simulink model "Model_14Bus_Microgrid_R2018"  (R2018b)
settings: Solver=ode23tb  StartTime=0.0  StopTime=0.35  MaxStep=1e-2  RelTol=1e-3
InitFcn:
  | Set_parameters_R2018
StopFcn:
  | Save_Data;
  | Graphics;
values from neighbouring files (symbols this model uses):
  Clink = Ceq*2    (= 0.217013888889)    [Set_parameters_R2017b.m]    (also in Set_parameters_R2018.m)
  dis1 = 0.15    [Set_parameters_R2017b.m]    (also in Set_parameters_R2018.m)
  dis10 = 6    [Set_parameters_R2017b.m]    (also in Set_parameters_R2018.m)
  dis11 = 3    [Set_parameters_R2017b.m]    (also in Set_parameters_R2018.m)
  dis12 = 6    [Set_parameters_R2017b.m]    (also in Set_parameters_R2018.m)
  dis13 = 3    [Set_parameters_R2017b.m]    (also in Set_parameters_R2018.m)
  dis14 = 2    [Set_parameters_R2017b.m]    (also in Set_parameters_R2018.m)
  dis2 = 0.2    [Set_parameters_R2017b.m]    (also in Set_parameters_R2018.m)
  dis3 = 0.15    [Set_parameters_R2017b.m]    (also in Set_parameters_R2018.m)
  dis4 = 0.4    [Set_parameters_R2017b.m]    (also in Set_parameters_R2018.m)
  dis5 = 0.4    [Set_parameters_R2017b.m]    (also in Set_parameters_R2018.m)
  dis6 = 0.4    [Set_parameters_R2017b.m]    (also in Set_parameters_R2018.m)
  dis7 = 0.1    [Set_parameters_R2017b.m]    (also in Set_parameters_R2018.m)
  dis8 = 2    [Set_parameters_R2017b.m]    (also in Set_parameters_R2018.m)
  dis9 = 6    [Set_parameters_R2017b.m]    (also in Set_parameters_R2018.m)
  Fc = 33 * Fnom    (= 1980)    [Set_parameters_R2017b.m]    (also in Set_parameters_R2018.m)
  Fnom = 60    [Main_DC_MG.m]    (also in Set_parameters_R2017b.m; Set_parameters_R2018.m)
  Increment_MPPT = 0.01    [Set_parameters_R2017b.m]    (also in Set_parameters_R2018.m)
  Ki_Ireg = 20    [Set_parameters_R2017b.m]    (also in Set_parameters_R2018.m)
  Ki_VDCreg = 400    [Set_parameters_R2017b.m]    (also in Set_parameters_R2018.m)
  Kp_Ireg = 0.3    [Set_parameters_R2017b.m]    (also in Set_parameters_R2018.m)
  Kp_VDCreg = 2    [Set_parameters_R2017b.m]    (also in Set_parameters_R2018.m)
  LimitL_Ireg = -1.5    [Set_parameters_R2017b.m]    (also in Set_parameters_R2018.m)
  LimitL_VDCreg = -1.5    [Set_parameters_R2017b.m]    (also in Set_parameters_R2018.m)
  Limits_MPPT = [ 583 357 ]    [Set_parameters_R2017b.m]    (also in Set_parameters_R2018.m)
  LimitU_Ireg = 1.5    [Set_parameters_R2017b.m]    (also in Set_parameters_R2018.m)
  LimitU_VDCreg = 1.5    [Set_parameters_R2017b.m]    (also in Set_parameters_R2018.m)
  P_Load_2 = S_Load_2* PF_Load_2    (= 36000)    [Set_parameters_R2017b.m]    (also in Set_parameters_R2018.m)
  P_Load_3 = S_Load_3* PF_Load_3    (= 25500)    [Set_parameters_R2017b.m]    (also in Set_parameters_R2018.m)
  Pnom = 1e6    (= 1000000)    [Set_parameters_R2017b.m]    (also in Set_parameters_R2018.m)
  Pnom_T1 = 1.5e6    (= 1500000)    [Set_parameters_R2017b.m]    (also in Set_parameters_R2018.m)
  Pnom_T2 = 1.5e6    (= 1500000)    [Set_parameters_R2017b.m]    (also in Set_parameters_R2018.m)
  Pnom_T3 = 4e6    (= 4000000)    [Set_parameters_R2017b.m]    (also in Set_parameters_R2018.m)
  Pnom_xfo = Pnom    (= 1000000)    [Set_parameters_R2017b.m]    (also in Set_parameters_R2018.m)
  Ql_Load_2 = S_Load_2 * sin(acos(PF_Load_2))    [Set_parameters_R2017b.m]    (also in Set_parameters_R2018.m)
  Ql_Load_3 = S_Load_3 * sin(acos(PF_Load_3))    [Set_parameters_R2017b.m]    (also in Set_parameters_R2018.m)
  R_Load_9 = (Vnom_prim * 1.35)^2 / P_Load_9    (= 1084.6153125)    [Set_parameters_R2017b.m]    (also in Set_parameters_R2018.m)
  R_Load_DC = Vnom_DC^2/ P_Load_DC    (= 45)    [Main_DC_MG.m]    (also in Set_parameters_R2017b.m; Set_parameters_R2018.m)
  Rl = 0.394    [Set_parameters_R2017b.m]    (also in Set_parameters_R2018.m)
  Rls = 0.198    [Set_parameters_R2017b.m]    (also in Set_parameters_R2018.m)
  Ts = Ts_Power    (= 5.05050505051e-06)    [Main_DC_MG.m]    (also in Set_parameters_R2017b.m; Set_parameters_R2018.m)
  Ts_Control = 10*Ts_Power    (= 5.05050505051e-05)    [Main_DC_MG.m]    (also in Set_parameters_R2017b.m; Set_parameters_R2018.m)
  Ts_Power = 1/(33*Fnom)/100    (= 5.05050505051e-06)    [Main_DC_MG.m]    (also in Set_parameters_R2017b.m; Set_parameters_R2018.m)
  V1_LL_T3 = 69e3    (= 69000)    [Set_parameters_R2017b.m]    (also in Set_parameters_R2018.m)
  Vf = 0    [Set_parameters_R2017b.m]    (also in Set_parameters_R2018.m)
  Vfd = 0    [Set_parameters_R2017b.m]    (also in Set_parameters_R2018.m)
  Vnom_DC = 300    [Main_DC_MG.m]    (also in Set_parameters_R2017b.m; Set_parameters_R2018.m)
  Vnom_dc = 480    [Set_parameters_R2017b.m]    (also in Set_parameters_R2018.m)
  Vnom_Diesel = 2.4e3    (= 2400)    [Set_parameters_R2017b.m]    (also in Set_parameters_R2018.m)
  Vnom_prim = 13.8e3    (= 13800)    [Set_parameters_R2017b.m]    (also in Set_parameters_R2018.m)
  Vnom_sec = 220    [Set_parameters_R2017b.m]    (also in Set_parameters_R2018.m)
  Vnom_ter_AC_DC = 150    [Set_parameters_R2017b.m]    (also in Set_parameters_R2018.m)
  Xl = 0.1168    [Set_parameters_R2017b.m]    (also in Set_parameters_R2018.m)
  Xls = 0.1089    [Set_parameters_R2017b.m]    (also in Set_parameters_R2018.m)
undefined symbols (not defined in the file or in its folder): D1, Delta, Hydride, Ion, Lithium, max_min, Metal, Nickel, RL, RLff, sigbuilder_block
libraries: powerlib x202, powerlib_meascontrol x152, simulink x14, powerlib_extras x14, electricdrivelib x4, re_lib x2
(part 6 of 10)

== system Model_14Bus_Microgrid_R2018/Bus_7/Power Factor Block1 ==
  Vabc : Inport
  Iabc : Inport  Port=2
  Complex to Magnitude-Angle : ComplexToMagnitudeAngle
  Conv pu2 : Gain  Gain=sqrt (3) /Vnom_prim  SaturateOnIntegerOverflow=on  OutDataTypeStr=Inherit: Same as input  ParamDataTypeStr=Inherit: Same as input
  Mux : Mux  Inputs=2
  Mux1 : Mux  Inputs=2
  Power : powerlib_meascontrol/Measurements/Power  Freq=Freq  Vinit=Vinit  Iinit=Iinit  Ts=Ts
      settings: SourceProductName=Simscape Electrical
  RMS3 : powerlib_meascontrol/Measurements/RMS  TrueRMS=on  Freq=60  RMSInit=0  Ts=0
      settings: SourceProductName=Simscape Electrical
  RMS4 : powerlib_meascontrol/Measurements/RMS  TrueRMS=on  Freq=60  RMSInit=0  Ts=0
      settings: SourceProductName=Simscape Electrical
  Real-Imag to Complex : RealImagToComplex
  Terminator : Terminator
  compara : Gain  SaturateOnIntegerOverflow=on  OutDataTypeStr=Inherit: Same as input  ParamDataTypeStr=Inherit: Same as input
  cos(theta) : Trigonometry  Operator=cos
  to Kw : Gain  Gain=1/1000
  to Kw1 : Gain  Gain=1/1000
  Pabc : Outport
  Qabc : Outport  Port=2
  Vabc y Vabc (rms) : Outport  Port=3
  Iabc y Iabc (rms) : Outport  Port=4
  "PFabc " : Outport  Port=5
  tag scope: P_abc_Bus7=global, Q_abc_Bus7=global, Vabc_LL_pu_Bus7=global
  wires:
  Complex to Magnitude-Angle/2 -> cos(theta)/1
  Real-Imag to Complex/1 -> Complex to Magnitude-Angle/1
  cos(theta)/1 -> "PFabc "/1
  Complex to Magnitude-Angle/1 -> Terminator/1
  Iabc/1 -> RMS4/1, compara/1, Power/2
  RMS4/1 -> Mux1/2
  Mux1/1 -> Iabc y Iabc (rms)/1
  Mux/1 -> Vabc y Vabc (rms)/1
  Vabc/1 -> Power/1, Mux/2, RMS3/1
  compara/1 -> Mux1/1
  Conv pu2/1 -> [Vabc_LL_pu_Bus7]
  RMS3/1 -> Conv pu2/1, Mux/1
  Power/2 -> Qabc/1, Real-Imag to Complex/2, to Kw/1
  Power/1 -> to Kw1/1, Pabc/1, Real-Imag to Complex/1
  to Kw/1 -> [Q_abc_Bus7]
  to Kw1/1 -> [P_abc_Bus7]

== system Model_14Bus_Microgrid_R2018/Bus_8      /PLL ==
  Vabc_LN_pu : Inport
  2pi60'1 : Constant  Value=2*pi*60
  2pi60'2 : Constant  Value=2*pi*60
  2pi60'3 : Constant  Value=2*pi*60
  Constant : Constant  Value=90
  Demux : Demux  Outputs=3
  Gain1 : Gain  Gain=180/pi  SaturateOnIntegerOverflow=on  OutDataTypeStr=Inherit: Same as input  ParamDataTypeStr=Inherit: Same as input
  Gain2 : Gain  Gain=180/pi  SaturateOnIntegerOverflow=on  OutDataTypeStr=Inherit: Same as input  ParamDataTypeStr=Inherit: Same as input
  Gain3 : Gain  Gain=180/pi  SaturateOnIntegerOverflow=on  OutDataTypeStr=Inherit: Same as input  ParamDataTypeStr=Inherit: Same as input
  Mux : Mux  Inputs=3
  Pll1 : Subsystem
  Pll2 : Subsystem
  Pll3 : Subsystem
  Sum : Sum  Inputs=|++
  delta_abc : Outport
  wires:
  Vabc_LN_pu/1 -> Demux/1
  Demux/1 -> Pll3/1(señal)
  2pi60'3/1 -> Pll3/2(w)
  Pll3/1(f cos (rad)) -> Gain1/1
  Demux/2 -> Pll1/1(señal)
  2pi60'1/1 -> Pll1/2(w)
  Gain2/1 -> Mux/2
  Demux/3 -> Pll2/1(señal)
  2pi60'2/1 -> Pll2/2(w)
  Pll2/1(f cos (rad)) -> Gain3/1
  Gain3/1 -> Mux/3
  Pll1/1(f cos (rad)) -> Gain2/1
  Mux/1 -> Sum/1
  Gain1/1 -> Mux/1
  Constant/1 -> Sum/2
  Sum/1 -> delta_abc/1

== system Model_14Bus_Microgrid_R2018/Bus_8      /Power Factor Block1 ==
  Vabc : Inport
  Iabc : Inport  Port=2
  Complex to Magnitude-Angle : ComplexToMagnitudeAngle
  Conv pu2 : Gain  Gain=sqrt (3) /Vnom_Diesel  SaturateOnIntegerOverflow=on  OutDataTypeStr=Inherit: Same as input  ParamDataTypeStr=Inherit: Same as input
  Gain : Gain  Gain=-1/1000
  Gain1 : Gain  Gain=-1/1000
  Mux : Mux  Inputs=2
  Mux1 : Mux  Inputs=2
  Power : powerlib_meascontrol/Measurements/Power  Freq=Freq  Vinit=Vinit  Iinit=Iinit  Ts=Ts
      settings: SourceProductName=Simscape Electrical
  RMS3 : powerlib_meascontrol/Measurements/RMS  TrueRMS=on  Freq=60  RMSInit=0  Ts=0
      settings: SourceProductName=Simscape Electrical
  RMS4 : powerlib_meascontrol/Measurements/RMS  TrueRMS=on  Freq=60  RMSInit=0  Ts=0
      settings: SourceProductName=Simscape Electrical
  Real-Imag to Complex : RealImagToComplex
  Terminator : Terminator
  compara : Gain  SaturateOnIntegerOverflow=on  OutDataTypeStr=Inherit: Same as input  ParamDataTypeStr=Inherit: Same as input
  cos(theta) : Trigonometry  Operator=cos
  Pabc : Outport
  Qabc : Outport  Port=2
  Vabc y Vabc (rms) : Outport  Port=3
  Iabc y Iabc (rms) : Outport  Port=4
  "PFabc " : Outport  Port=5
  tag scope: P_abc_Bus8=global, Q_abc_Bus8=global, Vabc_LL_pu_Bus8=global
  wires:
  Complex to Magnitude-Angle/2 -> cos(theta)/1
  Real-Imag to Complex/1 -> Complex to Magnitude-Angle/1
  cos(theta)/1 -> "PFabc "/1
  Complex to Magnitude-Angle/1 -> Terminator/1
  Iabc/1 -> RMS4/1, compara/1, Power/2
  RMS4/1 -> Mux1/2
  Mux1/1 -> Iabc y Iabc (rms)/1
  Mux/1 -> Vabc y Vabc (rms)/1
  Vabc/1 -> Power/1, Mux/2, RMS3/1
  compara/1 -> Mux1/1
  Conv pu2/1 -> [Vabc_LL_pu_Bus8]
  RMS3/1 -> Conv pu2/1, Mux/1
  Power/2 -> Qabc/1, Real-Imag to Complex/2, Gain/1
  Power/1 -> Gain1/1, Pabc/1, Real-Imag to Complex/1
  Gain/1 -> [Q_abc_Bus8]
  Gain1/1 -> [P_abc_Bus8]

== system Model_14Bus_Microgrid_R2018/Bus_9/PLL ==
  Vabc_LN_pu : Inport
  2pi60'1 : Constant  Value=2*pi*60
  2pi60'2 : Constant  Value=2*pi*60
  2pi60'3 : Constant  Value=2*pi*60
  Constant : Constant  Value=90
  Demux : Demux  Outputs=3
  Gain1 : Gain  Gain=180/pi  SaturateOnIntegerOverflow=on  OutDataTypeStr=Inherit: Same as input  ParamDataTypeStr=Inherit: Same as input
  Gain2 : Gain  Gain=180/pi  SaturateOnIntegerOverflow=on  OutDataTypeStr=Inherit: Same as input  ParamDataTypeStr=Inherit: Same as input
  Gain3 : Gain  Gain=180/pi  SaturateOnIntegerOverflow=on  OutDataTypeStr=Inherit: Same as input  ParamDataTypeStr=Inherit: Same as input
  Mux : Mux  Inputs=3
  Pll1 : Subsystem
  Pll2 : Subsystem
  Pll3 : Subsystem
  Sum : Sum  Inputs=|++
  delta_abc : Outport
  wires:
  Vabc_LN_pu/1 -> Demux/1
  Demux/1 -> Pll3/1(señal)
  2pi60'3/1 -> Pll3/2(w)
  Pll3/1(f cos (rad)) -> Gain1/1
  Demux/2 -> Pll1/1(señal)
  2pi60'1/1 -> Pll1/2(w)
  Gain2/1 -> Mux/2
  Demux/3 -> Pll2/1(señal)
  2pi60'2/1 -> Pll2/2(w)
  Pll2/1(f cos (rad)) -> Gain3/1
  Gain3/1 -> Mux/3
  Pll1/1(f cos (rad)) -> Gain2/1
  Mux/1 -> Sum/1
  Gain1/1 -> Mux/1
  Constant/1 -> Sum/2
  Sum/1 -> delta_abc/1

== system Model_14Bus_Microgrid_R2018/Bus_9/Power Factor Block1 ==
  Vabc : Inport
  Iabc : Inport  Port=2
  Complex to Magnitude-Angle : ComplexToMagnitudeAngle
  Conv pu2 : Gain  Gain=sqrt (3) /Vnom_prim  SaturateOnIntegerOverflow=on  OutDataTypeStr=Inherit: Same as input  ParamDataTypeStr=Inherit: Same as input
  Mux : Mux  Inputs=2
  Mux1 : Mux  Inputs=2
  Power : powerlib_meascontrol/Measurements/Power  Freq=Freq  Vinit=Vinit  Iinit=Iinit  Ts=Ts
      settings: SourceProductName=Simscape Electrical
  RMS3 : powerlib_meascontrol/Measurements/RMS  TrueRMS=on  Freq=60  RMSInit=0  Ts=0
      settings: SourceProductName=Simscape Electrical
  RMS4 : powerlib_meascontrol/Measurements/RMS  TrueRMS=on  Freq=60  RMSInit=0  Ts=0
      settings: SourceProductName=Simscape Electrical
  Real-Imag to Complex : RealImagToComplex
  Terminator : Terminator
  compara : Gain  SaturateOnIntegerOverflow=on  OutDataTypeStr=Inherit: Same as input  ParamDataTypeStr=Inherit: Same as input
  cos(theta) : Trigonometry  Operator=cos
  to Kw : Gain  Gain=1/1000
  to Kw1 : Gain  Gain=1/1000
  Pabc : Outport
  Qabc : Outport  Port=2
  Vabc y Vabc (rms) : Outport  Port=3
  Iabc y Iabc (rms) : Outport  Port=4
  "PFabc " : Outport  Port=5
  tag scope: P_abc_Bus9=global, Q_abc_Bus9=global, Vabc_LL_pu_Bus9=global
  wires:
  Complex to Magnitude-Angle/2 -> cos(theta)/1
  Real-Imag to Complex/1 -> Complex to Magnitude-Angle/1
  cos(theta)/1 -> "PFabc "/1
  Complex to Magnitude-Angle/1 -> Terminator/1
  Iabc/1 -> RMS4/1, compara/1, Power/2
  RMS4/1 -> Mux1/2
  Mux1/1 -> Iabc y Iabc (rms)/1
  Mux/1 -> Vabc y Vabc (rms)/1
  Vabc/1 -> Power/1, Mux/2, RMS3/1
  compara/1 -> Mux1/1
  RMS3/1 -> Conv pu2/1, Mux/1
  Conv pu2/1 -> [Vabc_LL_pu_Bus9]
  Power/2 -> Qabc/1, Real-Imag to Complex/2, to Kw/1
  Power/1 -> to Kw1/1, Pabc/1, Real-Imag to Complex/1
  to Kw/1 -> [Q_abc_Bus9]
  to Kw1/1 -> [P_abc_Bus9]

== system Model_14Bus_Microgrid_R2018/Bus_AC PV /PLL ==
  Vabc_LN_pu : Inport
  2pi60'1 : Constant  Value=2*pi*60
  2pi60'2 : Constant  Value=2*pi*60
  2pi60'3 : Constant  Value=2*pi*60
  Constant : Constant  Value=90
  Demux : Demux  Outputs=3
  Gain1 : Gain  Gain=180/pi  SaturateOnIntegerOverflow=on  OutDataTypeStr=Inherit: Same as input  ParamDataTypeStr=Inherit: Same as input
  Gain2 : Gain  Gain=180/pi  SaturateOnIntegerOverflow=on  OutDataTypeStr=Inherit: Same as input  ParamDataTypeStr=Inherit: Same as input
  Gain3 : Gain  Gain=180/pi  SaturateOnIntegerOverflow=on  OutDataTypeStr=Inherit: Same as input  ParamDataTypeStr=Inherit: Same as input
  Mux : Mux  Inputs=3
  Pll1 : Subsystem
  Pll2 : Subsystem
  Pll3 : Subsystem
  Sum : Sum  Inputs=|++
  delta_abc : Outport
  wires:
  Vabc_LN_pu/1 -> Demux/1
  Demux/1 -> Pll3/1(señal)
  2pi60'3/1 -> Pll3/2(w)
  Pll3/1(f cos (rad)) -> Gain1/1
  Demux/2 -> Pll1/1(señal)
  2pi60'1/1 -> Pll1/2(w)
  Gain2/1 -> Mux/2
  Demux/3 -> Pll2/1(señal)
  2pi60'2/1 -> Pll2/2(w)
  Pll2/1(f cos (rad)) -> Gain3/1
  Gain3/1 -> Mux/3
  Pll1/1(f cos (rad)) -> Gain2/1
  Mux/1 -> Sum/1
  Gain1/1 -> Mux/1
  Constant/1 -> Sum/2
  Sum/1 -> delta_abc/1

== system Model_14Bus_Microgrid_R2018/Bus_AC PV /Power Factor Block1 ==
  Vabc : Inport
  Iabc : Inport  Port=2
  Complex to Magnitude-Angle : ComplexToMagnitudeAngle
  Mux : Mux  Inputs=2
  Mux1 : Mux  Inputs=2
  Power : powerlib_meascontrol/Measurements/Power  Freq=Freq  Vinit=Vinit  Iinit=Iinit  Ts=Ts
      settings: SourceProductName=Simscape Electrical
  RMS3 : powerlib_meascontrol/Measurements/RMS  TrueRMS=on  Freq=60  RMSInit=0  Ts=0
      settings: SourceProductName=Simscape Electrical
  RMS4 : powerlib_meascontrol/Measurements/RMS  TrueRMS=on  Freq=60  RMSInit=0  Ts=0
      settings: SourceProductName=Simscape Electrical
  Real-Imag to Complex : RealImagToComplex
  Terminator : Terminator
  compara : Gain  SaturateOnIntegerOverflow=on  OutDataTypeStr=Inherit: Same as input  ParamDataTypeStr=Inherit: Same as input
  cos(theta) : Trigonometry  Operator=cos
  Pabc : Outport
  Qabc : Outport  Port=2
  Vabc y Vabc (rms) : Outport  Port=3
  Iabc y Iabc (rms) : Outport  Port=4
  "PFabc " : Outport  Port=5
  wires:
  Power/1 -> Pabc/1, Real-Imag to Complex/1
  Power/2 -> Qabc/1, Real-Imag to Complex/2
  Complex to Magnitude-Angle/2 -> cos(theta)/1
  Real-Imag to Complex/1 -> Complex to Magnitude-Angle/1
  cos(theta)/1 -> "PFabc "/1
  Complex to Magnitude-Angle/1 -> Terminator/1
  Iabc/1 -> RMS4/1, compara/1, Power/2
  RMS4/1 -> Mux1/2
  Mux1/1 -> Iabc y Iabc (rms)/1
  Mux/1 -> Vabc y Vabc (rms)/1
  Vabc/1 -> Power/1, Mux/2, RMS3/1
  compara/1 -> Mux1/1
  RMS3/1 -> Mux/1

== system Model_14Bus_Microgrid_R2018/Bus_AC//DC3/Battery system ==
  note: DC Bus
  note: Bettery
  "0 = Enable (Do it after transient, so that it does not calculate ripples during transient) 1 = Reset after every change in current reference" : Constant  Value=0
  Current Inst : Scope
  Current going to/ from the battery : Scope
  Display6 : Display
  Mean : powerlib_meascontrol/Measurements/Mean  Freq=10  Vinit=0  Ts=0
      settings: SourceProductName=Simscape Electrical
  Power : Product
  Power Bess : Scope
  Ripple Calculations : Subsystem
  Ripple in Boost : Display
  Ripple in Buck : Display
  Vbat : Scope
  Vdc : Scope
  to Kw : Gain  Gain=1/1000
  wires:
  to Kw/1 -> Display6/1, Power Bess/1
  Mean/1 -> Power/2
  Power/1 -> to Kw/1
  Ripple Calculations/1(Ripple in Buck) -> Ripple in Buck/1
  "0 = Enable (Do it after transient, so that it does not calculate ripples during transient) 1 = Reset after every change in current reference"/1 -> Ripple Calculations/2(Reset)
  Ripple Calculations/2(Ripple in Boost) -> Ripple in Boost/1
  [Idc_bus] -> Mean/1, Ripple Calculations/1(Signal), Current Inst/1
  [current] -> Current going to/ from the battery/1
  [Vdc_bus] -> Vdc/1, Power/1
  [Vdc_battery] -> Vbat/1

== system Model_14Bus_Microgrid_R2018/Bus_AC//DC3/PV system ==
  note: Bus DC
  note: PV
  Bus Selector : BusSelector  OutputSignals=V_PV,I_PV,I_diode,Irradiance (W/m2),Temperature (deg C)
  Current going to/ DC bus : Scope
  "P (kW) " : Display
      settings: Format=bank  Decimation=2000
  PV : Scope  NumInputPorts=3
  PV1 : Scope  NumInputPorts=5
  Pmean : Subsystem
  Vdc Boost : Display
      settings: Format=bank  Decimation=2000
  Vdc DC bus : Scope
  tag scope: I_PV=global, Idiode_PV=global, Ir=global, Temp=global, V_PV=global
  wires:
  [V_PV] -> PV/1  "V_PV"
  [I_PV] -> PV/2  "I_PV"
  [Idiode_PV] -> PV/3  "Idiode_PV"
  [m_PV] -> Bus Selector/1
  Bus Selector/1 -> [V_PV]  "<V_PV>"
  Bus Selector/2 -> [I_PV]  "<I_PV>"
  Bus Selector/4 -> [Ir]  "<Irradiance (W/m2)>"
  Bus Selector/3 -> [Idiode_PV]  "<I_diode>"
  Bus Selector/5 -> [Temp]  "<Temperature (deg C)>"
  [Temp] -> PV1/2  "Temp (deg. C)"
  [D] -> PV1/5  "Duty Cycle"
  Pmean/2(V) -> Vdc Boost/1, PV1/4  "Vmean (V)"
  [Ir] -> PV1/1  "Ir (W/m^2)"
  Pmean/1(P) -> "P (kW) "/1, PV1/3  "Pmean  (kW)"
  [I_DC_bus_PV] -> Current going to/ DC bus/1
  [V_DC_bus_PV] -> Vdc DC bus/1

== system Model_14Bus_Microgrid_R2018/Bus_AC//DC4/PLL ==
  Vabc_LN_pu : Inport
  2pi60'1 : Constant  Value=2*pi*60
  2pi60'2 : Constant  Value=2*pi*60
  2pi60'3 : Constant  Value=2*pi*60
  Constant : Constant  Value=90
  Demux : Demux  Outputs=3
  Gain1 : Gain  Gain=180/pi  SaturateOnIntegerOverflow=on  OutDataTypeStr=Inherit: Same as input  ParamDataTypeStr=Inherit: Same as input
  Gain2 : Gain  Gain=180/pi  SaturateOnIntegerOverflow=on  OutDataTypeStr=Inherit: Same as input  ParamDataTypeStr=Inherit: Same as input
  Gain3 : Gain  Gain=180/pi  SaturateOnIntegerOverflow=on  OutDataTypeStr=Inherit: Same as input  ParamDataTypeStr=Inherit: Same as input
  Mux : Mux  Inputs=3
  Pll1 : Subsystem
  Pll2 : Subsystem
  Pll3 : Subsystem
  Sum : Sum  Inputs=|++
  delta_abc : Outport
  wires:
  Vabc_LN_pu/1 -> Demux/1
  Demux/1 -> Pll3/1(señal)
  2pi60'3/1 -> Pll3/2(w)
  Pll3/1(f cos (rad)) -> Gain1/1
  Demux/2 -> Pll1/1(señal)
  2pi60'1/1 -> Pll1/2(w)
  Gain2/1 -> Mux/2
  Demux/3 -> Pll2/1(señal)
  2pi60'2/1 -> Pll2/2(w)
  Pll2/1(f cos (rad)) -> Gain3/1
  Gain3/1 -> Mux/3
  Pll1/1(f cos (rad)) -> Gain2/1
  Mux/1 -> Sum/1
  Gain1/1 -> Mux/1
  Constant/1 -> Sum/2
  Sum/1 -> delta_abc/1

== system Model_14Bus_Microgrid_R2018/Bus_AC//DC4/Power Factor Block1 ==
  Vabc : Inport
  Iabc : Inport  Port=2
  Complex to Magnitude-Angle : ComplexToMagnitudeAngle
  Mux : Mux  Inputs=2
  Mux1 : Mux  Inputs=2
  Power : powerlib_meascontrol/Measurements/Power  Freq=Freq  Vinit=Vinit  Iinit=Iinit  Ts=Ts
      settings: SourceProductName=Simscape Electrical
  RMS3 : powerlib_meascontrol/Measurements/RMS  TrueRMS=on  Freq=60  RMSInit=0  Ts=0
      settings: SourceProductName=Simscape Electrical
  RMS4 : powerlib_meascontrol/Measurements/RMS  TrueRMS=on  Freq=60  RMSInit=0  Ts=0
      settings: SourceProductName=Simscape Electrical
  Real-Imag to Complex : RealImagToComplex
  Terminator : Terminator
  compara : Gain  SaturateOnIntegerOverflow=on  OutDataTypeStr=Inherit: Same as input  ParamDataTypeStr=Inherit: Same as input
  cos(theta) : Trigonometry  Operator=cos
  Pabc : Outport
  Qabc : Outport  Port=2
  Vabc y Vabc (rms) : Outport  Port=3
  Iabc y Iabc (rms) : Outport  Port=4
  "PFabc " : Outport  Port=5
  wires:
  Power/1 -> Pabc/1, Real-Imag to Complex/1
  Power/2 -> Qabc/1, Real-Imag to Complex/2
  Complex to Magnitude-Angle/2 -> cos(theta)/1
  Real-Imag to Complex/1 -> Complex to Magnitude-Angle/1
  cos(theta)/1 -> "PFabc "/1
  Complex to Magnitude-Angle/1 -> Terminator/1
  Iabc/1 -> RMS4/1, compara/1, Power/2
  RMS4/1 -> Mux1/2
  Mux1/1 -> Iabc y Iabc (rms)/1
  Mux/1 -> Vabc y Vabc (rms)/1
  Vabc/1 -> Power/1, Mux/2, RMS3/1
  compara/1 -> Mux1/1
  RMS3/1 -> Mux/1

== system Model_14Bus_Microgrid_R2018/Bus_AC//DC5/PLL ==
  Vabc_LN_pu : Inport
  2pi60'1 : Constant  Value=2*pi*60
  2pi60'2 : Constant  Value=2*pi*60
  2pi60'3 : Constant  Value=2*pi*60
  Constant : Constant  Value=90
  Demux : Demux  Outputs=3
  Gain1 : Gain  Gain=180/pi  SaturateOnIntegerOverflow=on  OutDataTypeStr=Inherit: Same as input  ParamDataTypeStr=Inherit: Same as input
  Gain2 : Gain  Gain=180/pi  SaturateOnIntegerOverflow=on  OutDataTypeStr=Inherit: Same as input  ParamDataTypeStr=Inherit: Same as input
  Gain3 : Gain  Gain=180/pi  SaturateOnIntegerOverflow=on  OutDataTypeStr=Inherit: Same as input  ParamDataTypeStr=Inherit: Same as input
  Mux : Mux  Inputs=3
  Pll1 : Subsystem
  Pll2 : Subsystem
  Pll3 : Subsystem
  Sum : Sum  Inputs=|++
  delta_abc : Outport
  wires:
  Vabc_LN_pu/1 -> Demux/1
  Demux/1 -> Pll3/1(señal)
  2pi60'3/1 -> Pll3/2(w)
  Pll3/1(f cos (rad)) -> Gain1/1
  Demux/2 -> Pll1/1(señal)
  2pi60'1/1 -> Pll1/2(w)
  Gain2/1 -> Mux/2
  Demux/3 -> Pll2/1(señal)
  2pi60'2/1 -> Pll2/2(w)
  Pll2/1(f cos (rad)) -> Gain3/1
  Gain3/1 -> Mux/3
  Pll1/1(f cos (rad)) -> Gain2/1
  Mux/1 -> Sum/1
  Gain1/1 -> Mux/1
  Constant/1 -> Sum/2
  Sum/1 -> delta_abc/1

== system Model_14Bus_Microgrid_R2018/Bus_AC//DC5/Power Factor Block1 ==
  Vabc : Inport
  Iabc : Inport  Port=2
  Complex to Magnitude-Angle : ComplexToMagnitudeAngle
  Mux : Mux  Inputs=2
  Mux1 : Mux  Inputs=2
  Power : powerlib_meascontrol/Measurements/Power  Freq=Freq  Vinit=Vinit  Iinit=Iinit  Ts=Ts
      settings: SourceProductName=Simscape Electrical
  RMS3 : powerlib_meascontrol/Measurements/RMS  TrueRMS=on  Freq=60  RMSInit=0  Ts=0
      settings: SourceProductName=Simscape Electrical
  RMS4 : powerlib_meascontrol/Measurements/RMS  TrueRMS=on  Freq=60  RMSInit=0  Ts=0
      settings: SourceProductName=Simscape Electrical
  Real-Imag to Complex : RealImagToComplex
  Terminator : Terminator
  compara : Gain  SaturateOnIntegerOverflow=on  OutDataTypeStr=Inherit: Same as input  ParamDataTypeStr=Inherit: Same as input
  cos(theta) : Trigonometry  Operator=cos
  Pabc : Outport
  Qabc : Outport  Port=2
  Vabc y Vabc (rms) : Outport  Port=3
  Iabc y Iabc (rms) : Outport  Port=4
  "PFabc " : Outport  Port=5
  wires:
  Power/1 -> Pabc/1, Real-Imag to Complex/1
  Power/2 -> Qabc/1, Real-Imag to Complex/2
  Complex to Magnitude-Angle/2 -> cos(theta)/1
  Real-Imag to Complex/1 -> Complex to Magnitude-Angle/1
  cos(theta)/1 -> "PFabc "/1
  Complex to Magnitude-Angle/1 -> Terminator/1
  Iabc/1 -> RMS4/1, compara/1, Power/2
  RMS4/1 -> Mux1/2
  Mux1/1 -> Iabc y Iabc (rms)/1
  Mux/1 -> Vabc y Vabc (rms)/1
  Vabc/1 -> Power/1, Mux/2, RMS3/1
  compara/1 -> Mux1/1
  RMS3/1 -> Mux/1

== system Model_14Bus_Microgrid_R2018/Bus_slack /PLL ==
  Vabc_LN_pu : Inport
  2pi60'1 : Constant  Value=2*pi*60
  2pi60'2 : Constant  Value=2*pi*60
  2pi60'3 : Constant  Value=2*pi*60
  Constant : Constant  Value=90
  Demux : Demux  Outputs=3
  Gain1 : Gain  Gain=180/pi  SaturateOnIntegerOverflow=on  OutDataTypeStr=Inherit: Same as input  ParamDataTypeStr=Inherit: Same as input
  Gain2 : Gain  Gain=180/pi  SaturateOnIntegerOverflow=on  OutDataTypeStr=Inherit: Same as input  ParamDataTypeStr=Inherit: Same as input
  Gain3 : Gain  Gain=180/pi  SaturateOnIntegerOverflow=on  OutDataTypeStr=Inherit: Same as input  ParamDataTypeStr=Inherit: Same as input
  Mux : Mux  Inputs=3
  Pll1 : Subsystem
  Pll2 : Subsystem
  Pll3 : Subsystem
  Sum : Sum  Inputs=|++
  delta_abc : Outport
  wires:
  Vabc_LN_pu/1 -> Demux/1
  Demux/1 -> Pll3/1(señal)
  2pi60'3/1 -> Pll3/2(w)
  Pll3/1(f cos (rad)) -> Gain1/1
  Demux/2 -> Pll1/1(señal)
  2pi60'1/1 -> Pll1/2(w)
  Gain2/1 -> Mux/2
  Demux/3 -> Pll2/1(señal)
  2pi60'2/1 -> Pll2/2(w)
  Pll2/1(f cos (rad)) -> Gain3/1
  Gain3/1 -> Mux/3
  Pll1/1(f cos (rad)) -> Gain2/1
  Mux/1 -> Sum/1
  Gain1/1 -> Mux/1
  Constant/1 -> Sum/2
  Sum/1 -> delta_abc/1

== system Model_14Bus_Microgrid_R2018/Bus_slack /Power Factor Block1 ==
  Vabc : Inport
  Iabc : Inport  Port=2
  Complex to Magnitude-Angle : ComplexToMagnitudeAngle
  Conv pu2 : Gain  Gain=sqrt (3) /Vnom_prim  SaturateOnIntegerOverflow=on  OutDataTypeStr=Inherit: Same as input  ParamDataTypeStr=Inherit: Same as input
  Gain : Gain  Gain=-1/1000
  Gain1 : Gain  Gain=-1/1000
  Mux : Mux  Inputs=2
  Mux1 : Mux  Inputs=2
  Power : powerlib_meascontrol/Measurements/Power  Freq=Freq  Vinit=Vinit  Iinit=Iinit  Ts=Ts
      settings: SourceProductName=Simscape Electrical
  RMS3 : powerlib_meascontrol/Measurements/RMS  TrueRMS=on  Freq=60  RMSInit=0  Ts=0
      settings: SourceProductName=Simscape Electrical
  RMS4 : powerlib_meascontrol/Measurements/RMS  TrueRMS=on  Freq=60  RMSInit=0  Ts=0
      settings: SourceProductName=Simscape Electrical
  Real-Imag to Complex : RealImagToComplex
  Terminator : Terminator
  compara : Gain  SaturateOnIntegerOverflow=on  OutDataTypeStr=Inherit: Same as input  ParamDataTypeStr=Inherit: Same as input
  cos(theta) : Trigonometry  Operator=cos
  Pabc : Outport
  Qabc : Outport  Port=2
  Vabc y Vabc (rms) : Outport  Port=3
  Iabc y Iabc (rms) : Outport  Port=4
  "PFabc " : Outport  Port=5
  tag scope: P_abc_Bus13=global, Q_abc_Bus13=global, Vabc_LL_pu_Bus13=global
  wires:
  Complex to Magnitude-Angle/2 -> cos(theta)/1
  Real-Imag to Complex/1 -> Complex to Magnitude-Angle/1
  cos(theta)/1 -> "PFabc "/1
  Complex to Magnitude-Angle/1 -> Terminator/1
  Iabc/1 -> RMS4/1, compara/1, Power/2
  RMS4/1 -> Mux1/2
  Mux1/1 -> Iabc y Iabc (rms)/1
  Mux/1 -> Vabc y Vabc (rms)/1
  Vabc/1 -> Power/1, Mux/2, RMS3/1
  compara/1 -> Mux1/1
  RMS3/1 -> Conv pu2/1, Mux/1
  Conv pu2/1 -> [Vabc_LL_pu_Bus13]
  Power/1 -> Gain/1, Pabc/1, Real-Imag to Complex/1
  Power/2 -> Qabc/1, Real-Imag to Complex/2, Gain1/1
  Gain1/1 -> [Q_abc_Bus13]
  Gain/1 -> [P_abc_Bus13]

== system Model_14Bus_Microgrid_R2018/Control measurement/measurement ==
  Ground4 : powerlib/Elements/Ground  LConnTagsString=a
      settings: SourceProductName=Simscape Electrical
  Mux1 : Mux  Inputs=3
  Mux2 : Mux  Inputs=3
  Mux7 : Mux  Inputs=3
  Vab : powerlib/Measurements/Voltage Measurement  Tag=PoWeRsYsTeMmEaSuReMeNt  PhasorSimulation=off  OutputType=Magnitude  PSBequivalent=0
      settings: SourceProductName=Simscape Electrical
  Vab{1..3,5} (4 alike) : powerlib_extras/Discrete Measurements/Discrete  RMS value  Freq=60  Mag_Init=0  Ts=Ts_Power
  Vbc : powerlib/Measurements/Voltage Measurement  Tag=PoWeRsYsTeMmEaSuReMeNt  PhasorSimulation=off  OutputType=Magnitude  PSBequivalent=0
      settings: SourceProductName=Simscape Electrical
  Vca : powerlib/Measurements/Voltage Measurement  Tag=PoWeRsYsTeMmEaSuReMeNt  PhasorSimulation=off  OutputType=Magnitude  PSBequivalent=0
      settings: SourceProductName=Simscape Electrical
  a : powerlib/Measurements/Voltage Measurement  Tag=PoWeRsYsTeMmEaSuReMeNt  PhasorSimulation=off  OutputType=Magnitude  PSBequivalent=0
      settings: SourceProductName=Simscape Electrical
  b : powerlib/Measurements/Voltage Measurement  Tag=PoWeRsYsTeMmEaSuReMeNt  PhasorSimulation=off  OutputType=Magnitude  PSBequivalent=0
      settings: SourceProductName=Simscape Electrical
  c : powerlib/Measurements/Voltage Measurement  Tag=PoWeRsYsTeMmEaSuReMeNt  PhasorSimulation=off  OutputType=Magnitude  PSBequivalent=0
      settings: SourceProductName=Simscape Electrical
  A : PMIOPort  Side=Left
  B : PMIOPort  Port=2  Side=Left
  C : PMIOPort  Port=3  Side=Left
  Vph : Outport
  VL-L : Outport  Port=2
  VL-L_rms : Outport  Port=3
  Vph_rms : Outport  Port=4
  wires:
  a/1 -> Mux7/1, Vab5/1
  b/1 -> Mux7/2, Vab1/1
  c/1 -> Mux7/3, Vab2/1
  Mux7/1 -> Vph/1
  Vab/1 -> Mux1/1
  Vbc/1 -> Mux1/2
  Vca/1 -> Mux1/3
  Mux1/1 -> Vab3/1, VL-L/1
  Vab5/1 -> Mux2/1
  Vab1/1 -> Mux2/2
  Vab2/1 -> Mux2/3
  Mux2/1 -> Vph_rms/1
  Vab3/1 -> VL-L_rms/1
  connections:
  Ground4/LConn1 -- c/LConn2 -- b/LConn2 -- a/LConn2
  A/RConn1 -- a/LConn1 -- Vab/LConn1 -- Vca/LConn2
  B/RConn1 -- b/LConn1 -- Vab/LConn2 -- Vbc/LConn1
  C/RConn1 -- c/LConn1 -- Vbc/LConn2 -- Vca/LConn1

== system Model_14Bus_Microgrid_R2018/Control measurement2/measurement2 ==
  Ground4 : powerlib/Elements/Ground  LConnTagsString=a
      settings: SourceProductName=Simscape Electrical
  Mux1 : Mux  Inputs=3
  Mux2 : Mux  Inputs=3
  Mux7 : Mux  Inputs=3
  Vab : powerlib/Measurements/Voltage Measurement  Tag=PoWeRsYsTeMmEaSuReMeNt  PhasorSimulation=off  OutputType=Magnitude  PSBequivalent=0
      settings: SourceProductName=Simscape Electrical
  Vab{1..3,5} (4 alike) : powerlib_extras/Discrete Measurements/Discrete  RMS value  Freq=60  Mag_Init=0  Ts=Ts_Power
  Vbc : powerlib/Measurements/Voltage Measurement  Tag=PoWeRsYsTeMmEaSuReMeNt  PhasorSimulation=off  OutputType=Magnitude  PSBequivalent=0
      settings: SourceProductName=Simscape Electrical
  Vca : powerlib/Measurements/Voltage Measurement  Tag=PoWeRsYsTeMmEaSuReMeNt  PhasorSimulation=off  OutputType=Magnitude  PSBequivalent=0
      settings: SourceProductName=Simscape Electrical
  a : powerlib/Measurements/Voltage Measurement  Tag=PoWeRsYsTeMmEaSuReMeNt  PhasorSimulation=off  OutputType=Magnitude  PSBequivalent=0
      settings: SourceProductName=Simscape Electrical
  b : powerlib/Measurements/Voltage Measurement  Tag=PoWeRsYsTeMmEaSuReMeNt  PhasorSimulation=off  OutputType=Magnitude  PSBequivalent=0
      settings: SourceProductName=Simscape Electrical
  c : powerlib/Measurements/Voltage Measurement  Tag=PoWeRsYsTeMmEaSuReMeNt  PhasorSimulation=off  OutputType=Magnitude  PSBequivalent=0
      settings: SourceProductName=Simscape Electrical
  A : PMIOPort  Side=Left
  B : PMIOPort  Port=2  Side=Left
  C : PMIOPort  Port=3  Side=Left
  Vph : Outport
  VL-L : Outport  Port=2
  VL-L_rms : Outport  Port=3
  Vph_rms : Outport  Port=4
  wires:
  a/1 -> Mux7/1, Vab5/1
  b/1 -> Mux7/2, Vab1/1
  c/1 -> Mux7/3, Vab2/1
  Mux7/1 -> Vph/1
  Vab/1 -> Mux1/1
  Vbc/1 -> Mux1/2
  Vca/1 -> Mux1/3
  Mux1/1 -> Vab3/1, VL-L/1
  Vab5/1 -> Mux2/1
  Vab1/1 -> Mux2/2
  Vab2/1 -> Mux2/3
  Mux2/1 -> Vph_rms/1
  Vab3/1 -> VL-L_rms/1
  connections:
  Ground4/LConn1 -- c/LConn2 -- b/LConn2 -- a/LConn2
  A/RConn1 -- a/LConn1 -- Vab/LConn1 -- Vca/LConn2
  B/RConn1 -- b/LConn1 -- Vab/LConn2 -- Vbc/LConn1
  C/RConn1 -- c/LConn1 -- Vbc/LConn2 -- Vca/LConn1

== system Model_14Bus_Microgrid_R2018/DATA  ADQUISITION/Delta_abc ==
  Mux3 : Mux  Inputs=14
  f3 : ToWorkspace  VariableName=ang_abc  SaveFormat=Timeseries  SampleTime=-1
  wires:
  [delta_abc_Bus10] -> Mux3/10
  [delta_abc_Bus4] -> Mux3/4
  [delta_abc_Bus7] -> Mux3/7
  [delta_abc_Bus8] -> Mux3/8
  [delta_abc_Bus11] -> Mux3/11
  [delta_abc_Bus5] -> Mux3/5
  [delta_abc_Bus9] -> Mux3/9
  [delta_abc_Bus2] -> Mux3/2
  [delta_abc_Bus1] -> Mux3/1
  [delta_abc_Bus12] -> Mux3/12
  [delta_abc_Bus14] -> Mux3/14
  Mux3/1 -> f3/1
  [delta_abc_Bus6] -> Mux3/6
  [delta_abc_Bus13] -> Mux3/13
  [delta_abc_Bus3] -> Mux3/3

== system Model_14Bus_Microgrid_R2018/DATA  ADQUISITION/PF_abc ==
  Mux2 : Mux  Inputs=14
  f3 : ToWorkspace  VariableName=PF_abc  SaveFormat=Timeseries  SampleTime=-1
  wires:
  [PFabc_Bus2] -> Mux2/2
  [PFabc_Bus4] -> Mux2/4
  [PFabc_Bus1] -> Mux2/1
  [PFabc_Bus6] -> Mux2/6
  Mux2/1 -> f3/1
  [PFabc_Bus5] -> Mux2/5
  [PFabc_Bus14] -> Mux2/14
  [PFabc_Bus8] -> Mux2/8
  [PFabc_Bus9] -> Mux2/9
  [PFabc_Bus7] -> Mux2/7
  [PFabc_Bus11] -> Mux2/11
  [PFabc_Bus13] -> Mux2/13
  [PFabc_Bus10] -> Mux2/10
  [PFabc_Bus3] -> Mux2/3
  [PFabc_Bus12] -> Mux2/12

== system Model_14Bus_Microgrid_R2018/DATA  ADQUISITION/P_abc ==
  Mux : Mux  Inputs=15
  f1 : ToWorkspace  VariableName=P_abc  SaveFormat=Timeseries  SampleTime=-1
  wires:
  [P_abc_Bus1] -> Mux/1
  [P_abc_Bus3] -> Mux/3
  [P_abc_Bus2] -> Mux/2
  [P_abc_Bus13] -> Mux/13
  Mux/1 -> f1/1
  [P_abc_Bus12] -> Mux/12
  [P_abc_Bus9] -> Mux/9
  [P_abc_Bus8] -> Mux/8
  [P_abc_Bus10] -> Mux/10
  [P_abc_Bus11] -> Mux/11
  [P_abc_Bus7] -> Mux/7
  [P_abc_Bus4] -> Mux/4
  [P_abc_Bus14] -> Mux/14
  [P_abc_Bus5] -> Mux/5
  [P_BusDC] -> Mux/15
  [P_abc_Bus6] -> Mux/6

== system Model_14Bus_Microgrid_R2018/DATA  ADQUISITION/Power_Losses_abc ==
  Mux : Mux  Inputs=14
  f2 : ToWorkspace  VariableName=Power_Losse_abc  SaveFormat=Timeseries  SampleTime=-1
  wires:
  [Power_Losse_abc_L12] -> Mux/12
  [Power_Losse_abc_L10] -> Mux/10
  [Power_Losse_abc_L13] -> Mux/13
  [Power_Losse_abc_L1] -> Mux/1
  Mux/1 -> f2/1
  [Power_Losse_abc_L2] -> Mux/2
  [Power_Losse_abc_L3] -> Mux/3
  [Power_Losse_abc_L4] -> Mux/4
  [Power_Losse_abc_L5] -> Mux/5
  [Power_Losse_abc_L14] -> Mux/14
  [Power_Losse_abc_L9] -> Mux/9
  [Power_Losse_abc_L6] -> Mux/6
  [Power_Losse_abc_L8] -> Mux/8
  [Power_Losse_abc_L11] -> Mux/11
  [Power_Losse_abc_L7] -> Mux/7

== system Model_14Bus_Microgrid_R2018/DATA  ADQUISITION/Q_abc ==
  Mux2 : Mux  Inputs=14
  f2 : ToWorkspace  VariableName=Q_abc  SaveFormat=Timeseries  SampleTime=-1
  wires:
  Mux2/1 -> f2/1
  [Q_abc_Bus6] -> Mux2/6
  [Q_abc_Bus1] -> Mux2/1
  [Q_abc_Bus4] -> Mux2/4
  [Q_abc_Bus5] -> Mux2/5
  [Q_abc_Bus9] -> Mux2/9
  [Q_abc_Bus10] -> Mux2/10
  [Q_abc_Bus2] -> Mux2/2
  [Q_abc_Bus12] -> Mux2/12
  [Q_abc_Bus8] -> Mux2/8
  [Q_abc_Bus13] -> Mux2/13
  [Q_abc_Bus3] -> Mux2/3
  [Q_abc_Bus11] -> Mux2/11
  [Q_abc_Bus14] -> Mux2/14
  [Q_abc_Bus7] -> Mux2/7

== system Model_14Bus_Microgrid_R2018/DATA  ADQUISITION/THDv_abc ==
  Mux1 : Mux  Inputs=14
  f1 : ToWorkspace  VariableName=THDv_abc  SaveFormat=Timeseries  SampleTime=-1
  wires:
  [THDv_abc_Bus8] -> Mux1/8
  [THDv_abc_Bus5] -> Mux1/5
  [THDv_abc_Bus1] -> Mux1/1
  Mux1/1 -> f1/1
  [THDv_abc_Bus7] -> Mux1/7
  [THDv_abc_Bus11] -> Mux1/11
  [THDv_abc_Bus4] -> Mux1/4
  [THDv_abc_Bus9] -> Mux1/9
  [THDv_abc_Bus6] -> Mux1/6
  [THDv_abc_Bus14] -> Mux1/14
  [THDv_abc_Bus3] -> Mux1/3
  [THDv_abc_Bus2] -> Mux1/2
  [THDv_abc_Bus13] -> Mux1/13
  [THDv_abc_Bus10] -> Mux1/10
  [THDv_abc_Bus12] -> Mux1/12

== system Model_14Bus_Microgrid_R2018/DATA  ADQUISITION/VoltageLL_pu_abc ==
  Mux : Mux  Inputs=15
  f2 : ToWorkspace  VariableName=VoltageLL_pu_abc  SaveFormat=Timeseries  SampleTime=-1
  wires:
  [Vabc_LL_pu_Bus4] -> Mux/4
  [Vabc_LL_pu_Bus3] -> Mux/3
  [Vabc_LL_pu_Bus5] -> Mux/5
  Mux/1 -> f2/1
  [Vabc_LL_pu_Bus8] -> Mux/8
  [Vabc_LL_pu_Bus1] -> Mux/1
  [Vabc_LL_pu_Bus2] -> Mux/2
  [Vabc_LL_pu_Bus11] -> Mux/11
  [Vabc_LL_pu_Bus12] -> Mux/12
  [Vabc_LL_pu_Bus6] -> Mux/6
  [Vabc_LL_pu_Bus14] -> Mux/14
  [Vabc_LL_pu_Bus7] -> Mux/7
  [V_pu_BusDC] -> Mux/15
  [Vabc_LL_pu_Bus13] -> Mux/13
  [Vabc_LL_pu_Bus9] -> Mux/9
  [Vabc_LL_pu_Bus10] -> Mux/10

== system Model_14Bus_Microgrid_R2018/Grid Bi-directional converter AC //CD 2 Cascaded Topology/BESS Control (A) ==
  COMPARATOR 1 : RelationalOperator  Operator=<=  OutDataTypeStr=boolean  RndMeth=Nearest
  COMPARATOR 2 : RelationalOperator  Operator=<=  OutDataTypeStr=boolean  RndMeth=Nearest
  Goto1 : Goto  Commented=on  GotoTag=c2
  Logical Operator : Logic  Operator=NOT  AllPortsSameDT=off  OutDataTypeStr=boolean
  Logical Operator1 : Logic  Operator=NOT  AllPortsSameDT=off  OutDataTypeStr=boolean
  Subsystem : Subsystem
  Subsystem1 : Subsystem
  sa11 : Outport
  sap11 : Outport  Port=2
  sa22 : Outport  Port=3
  sap22 : Outport  Port=4
  wires:
  Subsystem/1(carrier) -> [c1]
  [c1] -> COMPARATOR 1/1
  [c1] -> COMPARATOR 2/1
  Subsystem/2(delayed carrier) -> Goto1/1
  [c3] -> COMPARATOR 2/2
  [c4] -> COMPARATOR 1/2
  COMPARATOR 2/1 -> sa11/1, Logical Operator/1
  COMPARATOR 1/1 -> sa22/1, Logical Operator1/1
  Logical Operator1/1 -> sap22/1
  Logical Operator/1 -> sap11/1
  Subsystem1/1(5*sin) -> [c3]
  Subsystem1/2(-5*sin) -> [c4]

== system Model_14Bus_Microgrid_R2018/Grid Bi-directional converter AC //CD 2 Cascaded Topology/BESS Control (B) ==
  note: .
  COMPARATOR 5 : RelationalOperator  Operator=<=  OutDataTypeStr=boolean  RndMeth=Nearest
  COMPARATOR 6 : RelationalOperator  Operator=<=  OutDataTypeStr=boolean  RndMeth=Nearest
  Goto13 : Goto  Commented=on  GotoTag=c22
  Logical Operator4 : Logic  Operator=NOT  AllPortsSameDT=off  OutDataTypeStr=boolean
  Logical Operator5 : Logic  Operator=NOT  AllPortsSameDT=off  OutDataTypeStr=boolean
  Subsystem2 : Subsystem
  Subsystem3 : Subsystem
  sb11 : Outport
  sbp11 : Outport  Port=2
  sb22 : Outport  Port=3
  sbp22 : Outport  Port=4
  wires:
  Subsystem2/2(delayed carrier) -> Goto13/1
  Subsystem2/1(carrier) -> [c11]
  [c11] -> COMPARATOR 6/1
  [c44] -> COMPARATOR 5/2
  [c11] -> COMPARATOR 5/1
  [c33] -> COMPARATOR 6/2
  COMPARATOR 5/1 -> sb22/1, Logical Operator5/1
  COMPARATOR 6/1 -> sb11/1, Logical Operator4/1
  Logical Operator4/1 -> sbp11/1
  Logical Operator5/1 -> sbp22/1
  Subsystem3/1(4.8*sin) -> [c33]
  Subsystem3/2(-4.8*sin) -> [c44]

== system Model_14Bus_Microgrid_R2018/Grid Bi-directional converter AC //CD 2 Cascaded Topology/BESS Control (C) ==
  COMPARATOR 10 : RelationalOperator  Operator=<=  OutDataTypeStr=boolean  RndMeth=Nearest
  COMPARATOR 9 : RelationalOperator  Operator=<=  OutDataTypeStr=boolean  RndMeth=Nearest
  Goto25 : Goto  Commented=on  GotoTag=c222
  Logical Operator8 : Logic  Operator=NOT  AllPortsSameDT=off  OutDataTypeStr=boolean
  Logical Operator9 : Logic  Operator=NOT  AllPortsSameDT=off  OutDataTypeStr=boolean
  Subsystem4 : Subsystem
  Subsystem5 : Subsystem
  sc11 : Outport
  scp11 : Outport  Port=2
  sc22 : Outport  Port=3
  scp22 : Outport  Port=4
  wires:
  Subsystem4/1(carrier) -> [c111]
  [c333] -> COMPARATOR 10/2
  Subsystem4/2(delayed carrier) -> Goto25/1
  [c111] -> COMPARATOR 9/1
  [c111] -> COMPARATOR 10/1
  COMPARATOR 10/1 -> sc11/1, Logical Operator8/1
  [c444] -> COMPARATOR 9/2
  COMPARATOR 9/1 -> sc22/1, Logical Operator9/1
  Logical Operator8/1 -> scp11/1
  Logical Operator9/1 -> scp22/1
  Subsystem5/1(4.8*sin) -> [c333]
  Subsystem5/2(-4.8*sin) -> [c444]

== system Model_14Bus_Microgrid_R2018/Grid Bi-directional Converter 1.1 300 (DC) // 150 V (AC) P_nom 3kW/Control of Inverter ==
  note: VL-L rms_1
  note: Primary control
  note: Control of Inverter
  Means : Inport
  Bus Selector : BusSelector  OutputSignals=signal1,signal2,signal3,signal4
  Discrete PWM Generator1 : Subsystem  AncestorBlock=|  DialogController=POWERSYS.PowerSysDialog  mask(Discrete PWM Generator){GeneratorMode=3-arm  bridge (6 pulses), Fc=4000, Ts=Ts_Power, Internal=off, mIndex=0.99, Freq=60, Phase=0}
      | powerlib_extras/Discrete 
      | Control Blocks/Discrete
      | PWM Generator
      mask prompts: GeneratorMode "Generator Mode"; Fc "Carrier frequency (Hz):"; Ts "Sample time:"; Internal "Internal generation of modulating signal(s)"; mIndex "Modulation index  (0<m<1) :"; Freq "Frequency of output voltage (Hz)"; Phase "Phase of output voltage (degrees)"
      mask help:
      | This discrete block generates pulses for carrier-based PWM (Pulse Width Modulation), self-commutated IGBTs,GTOs or FETs bridges.
      |
      | Depending on the number of bridge arms selected in the "Generator Mode" parameter, the block can be used either for single-phase or three-phase PWM control.
      mask init:
      | powericon('psbcallbacks',gcb,'Discrete PWM Generator');
      | if Freq==0
      |     Phase=90;
      | end
      | switch GeneratorMode
      | case 1,
      |     Internal_Phase=0;
      |    Signal_PortWidth=1;
      |    Select1_Elements=[1 2];
      |    Select1_PortWidth=2;
      |    Select3_Elements=[1 2];
      |    Select3_PortWidth=4;
      | case 2,
      |     Internal_Phase=0;
      |     Signal_PortWidth=1;
      |     Select1_Elements=[1 2];
      |     Select1_PortWidth=2;
      |     Select3_Elements=[1 2 3 4];
      |     Select3_PortWidth=4;
      | case 3,
      |     Internal_Phase=[0 -2*pi/3 2*pi/3];
      |     Signal_PortWidth=3;
      |     Select1_Elements=[1 4 2 5 3 6];
      |     Select1_PortWidth=6;
      |    Select3_Elements=[1 2 3 4 5 6];
      |    Select3_PortWidth=12;
      | case 4,
      |     Internal_Phase=[0 -2*pi/3 2*pi/3];
      |     Signal_PortWidth=3;
      |     Select1_Elements=[1 4 2 5 3 6];
      |     Select1_PortWidth=6;
      |    Select3_Elements=[1 2 3 4 5 6 7 8 9 10 11 12];
      |    Select3_PortWidth=12;
      | end
      | power_initmask();
      mask Help:
      | The output pulses are a vector (with values=0 or 1). Depending on the selected "Generator Mode", the output vector contains:
      | For a 1-arm  bridge: Two pulses. Pulse 1 is for the upper switch and pulse 2 is for the lower switch.
      | For a 2-arm  bridge: Four pulses. Pulses 1 and 3 are respectively for the upper switches of the first and second arm. Pulses 2 and 4 are for the lower switches.
      | For a 3-arm  bridge: Six pulses. Pulses 1,3 and 5 are respectively for the upper switches of the first,second and third arm. Pulses 2,4 and 6 are for the lower switches.
      | For double 3-arm bridges: Twelve pulses.The first six pulses (pulses 1 to 6) must be sent to the first 3-arm bridge and the last six (pulses 7 to 12) to the second 3-arm bridge.
      | 
      | By selecting "Internal generation" you can can control the modulation index m, frequency and phase of the output voltage  from the internal parameters (m, Freq and Phase). Otherwise, external signals are used for pulse generation. The width of the input vector must be 1 for single phase bridges ( 1-arm or 2-arm)  and 3 for 3-phase bridges  (single or double bridge).
      mask TypeOptions GeneratorMode: 1-arm  bridge (2 pulses) | 2-arm  bridge (4 pulses) | 3-arm  bridge (6 pulses) | Double 3-arm  bridges (12 pulses)
      mask Callback Internal: powericon('psbcallbacks',gcb,'Discrete PWM Generator',[]);
  MI Controller : Subsystem
  Unit Delay4 : UnitDelay  SampleTime=Ts_Power
  VL-L_1 : Scope  NumInputPorts=2
  Vph_abc : Scope
  Vph_rms_1 : Scope
  u / m : Scope
  Pulses : Outport
  wires:
  MI Controller/2(u / m) -> u / m/1
  Unit Delay4/1 -> Pulses/1
  Discrete PWM Generator1/1(Pulses) -> Unit Delay4/1
  Bus Selector/1 -> Vph_abc/1, MI Controller/1(Vabc)  "<signal1>"
  Bus Selector/2 -> VL-L_1/1  "<signal2>"
  Bus Selector/3 -> VL-L_1/2  "<signal3>"
  Bus Selector/4 -> Vph_rms_1/1  "<signal4>"
  Means/1 -> Bus Selector/1
  MI Controller/1(Vabc_inv) -> Discrete PWM Generator1/1(Uref)

== system Model_14Bus_Microgrid_R2018/Grid Bi-directional Converter 1.2 300 (DC) // 150 V (AC) P_nom 3kW/Control of Inverter ==
  note: VL-L rms_2
  note: Primary control
  note: Control of Inverter
  Means2 : Inport
  Bus Selector : BusSelector  OutputSignals=signal1,signal2,signal3,signal4
  Discrete PWM Generator1 : Subsystem  AncestorBlock=|  DialogController=POWERSYS.PowerSysDialog  mask(Discrete PWM Generator){GeneratorMode=3-arm  bridge (6 pulses), Fc=4000, Ts=Ts_Power, Internal=off, mIndex=0.99, Freq=60, Phase=0}
      | powerlib_extras/Discrete 
      | Control Blocks/Discrete
      | PWM Generator
      mask prompts: GeneratorMode "Generator Mode"; Fc "Carrier frequency (Hz):"; Ts "Sample time:"; Internal "Internal generation of modulating signal(s)"; mIndex "Modulation index  (0<m<1) :"; Freq "Frequency of output voltage (Hz)"; Phase "Phase of output voltage (degrees)"
      mask help:
      | This discrete block generates pulses for carrier-based PWM (Pulse Width Modulation), self-commutated IGBTs,GTOs or FETs bridges.
      |
      | Depending on the number of bridge arms selected in the "Generator Mode" parameter, the block can be used either for single-phase or three-phase PWM control.
      mask init: same as Model_14Bus_Microgrid_R2018/Grid Bi-directional Converter 1.1 300 (DC) // 150 V (AC) P_nom 3kW/Control of Inverter/Discrete PWM Generator1
      mask Help:
      | The output pulses are a vector (with values=0 or 1). Depending on the selected "Generator Mode", the output vector contains:
      | For a 1-arm  bridge: Two pulses. Pulse 1 is for the upper switch and pulse 2 is for the lower switch.
      | For a 2-arm  bridge: Four pulses. Pulses 1 and 3 are respectively for the upper switches of the first and second arm. Pulses 2 and 4 are for the lower switches.
      | For a 3-arm  bridge: Six pulses. Pulses 1,3 and 5 are respectively for the upper switches of the first,second and third arm. Pulses 2,4 and 6 are for the lower switches.
      | For double 3-arm bridges: Twelve pulses.The first six pulses (pulses 1 to 6) must be sent to the first 3-arm bridge and the last six (pulses 7 to 12) to the second 3-arm bridge.
      | 
      | By selecting "Internal generation" you can can control the modulation index m, frequency and phase of the output voltage  from the internal parameters (m, Freq and Phase). Otherwise, external signals are used for pulse generation. The width of the input vector must be 1 for single phase bridges ( 1-arm or 2-arm)  and 3 for 3-phase bridges  (single or double bridge).
      mask TypeOptions GeneratorMode: 1-arm  bridge (2 pulses) | 2-arm  bridge (4 pulses) | 3-arm  bridge (6 pulses) | Double 3-arm  bridges (12 pulses)
      mask Callback Internal: powericon('psbcallbacks',gcb,'Discrete PWM Generator',[]);
  MI Controller : Subsystem
  Unit Delay4 : UnitDelay  SampleTime=Ts_Power
  VL-L_2 : Scope  NumInputPorts=2
  Vph_rms_2 : Scope
  m2 : Scope
  m_2 : Scope
  Pulses : Outport
  wires:
  MI Controller/2(m) -> m_2/1
  Unit Delay4/1 -> Pulses/1
  Discrete PWM Generator1/1(Pulses) -> Unit Delay4/1
  MI Controller/1(Vabc_inv) -> Discrete PWM Generator1/1(Uref)
  Bus Selector/1 -> m2/1, MI Controller/1(Vabc)  "<signal1>"
  Bus Selector/2 -> VL-L_2/1  "<signal2>"
  Bus Selector/3 -> VL-L_2/2  "<signal3>"
  Bus Selector/4 -> Vph_rms_2/1  "<signal4>"
  Means2/1 -> Bus Selector/1

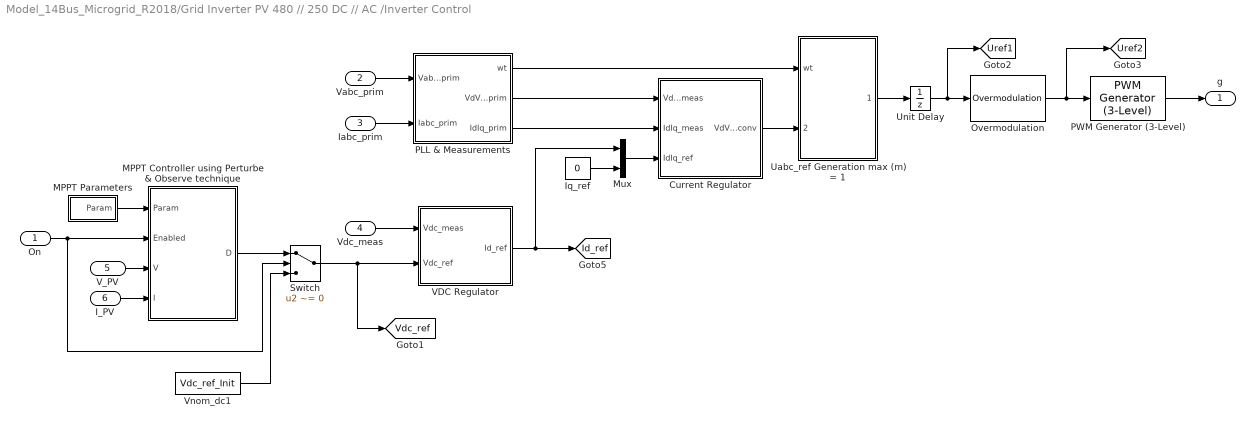
== system Model_14Bus_Microgrid_R2018/Grid Inverter PV 480 // 250 DC // AC /Inverter Control ==
  On : Inport  PortDimensions=1
  Vabc_prim : Inport  Port=2  PortDimensions=3
  Iabc_prim : Inport  Port=3  PortDimensions=3
  Vdc_meas : Inport  Port=4  PortDimensions=1
  V_PV : Inport  Port=5  PortDimensions=1
  I_PV : Inport  Port=6  PortDimensions=1
  Current Regulator : Subsystem
  Iq_ref : Constant  Value=0
  MPPT Parameters : Subsystem
  "MPPT Controller using Perturbe & Observe technique " : MATLAB Function  TreatAsAtomicUnit=on
  Mux : Mux  Inputs=2
  Overmodulation : powerlib_meascontrol/Pulse & Signal Generators/Overmodulation  OverModType=Flat top
      settings: SourceProductName=Simscape Electrical  SourceProductBaseCode=PS
  PLL & Measurements : Subsystem
  PWM Generator (3-Level) : powerlib_meascontrol/Pulse & Signal Generators/PWM Generator (3-Level)  ModulatorType=Three-phase bridge (12 pulses)  ModulatorMode=Unsynchronized  nF=27  Fc=Fc  ModulatingSignals=off  m=0.8  Freq=60  Phase=0  Ts=Ts_PWMgenerator
      settings: SourceProductName=Simscape Electrical  SourceProductBaseCode=PS
  Switch : Switch  Criteria=u2 ~= 0
  Uabc_ref Generation max (m) = 1 : Subsystem
  Unit Delay : UnitDelay  SampleTime=Ts_Control
  VDC Regulator : Subsystem
  Vnom_dc1 : Constant  Value=Vdc_ref_Init
  g : Outport
  tag scope: Id_ref=global, Uref1=global, Uref2=global, Vdc_ref=global
  wires:
  PLL & Measurements/1(wt) -> Uabc_ref Generation max (m) = 1/1(wt)
  Current Regulator/1(VdVq_conv) -> Uabc_ref Generation max (m) = 1/2(VdVq_conv)
  Iq_ref/1 -> Mux/2
  Mux/1 -> Current Regulator/3(IdIq_ref)
  PLL & Measurements/3(IdIq_prim) -> Current Regulator/2(IdIq_meas)
  PLL & Measurements/2(VdVq_prim) -> Current Regulator/1(VdVq_meas)
  Vabc_prim/1 -> PLL & Measurements/1(Vabc_prim)
  Iabc_prim/1 -> PLL & Measurements/2(Iabc_prim)
  PWM Generator (3-Level)/1 -> g/1
  Vdc_meas/1 -> VDC Regulator/1(Vdc_meas)
  VDC Regulator/1(Id_ref) -> [Id_ref], Mux/1
  V_PV/1 -> "MPPT Controller using Perturbe & Observe technique "/3(V)
  I_PV/1 -> "MPPT Controller using Perturbe & Observe technique "/4(I)
  MPPT Parameters/1(Param) -> "MPPT Controller using Perturbe & Observe technique "/1(Param)
  On/1 -> "MPPT Controller using Perturbe & Observe technique "/2(Enabled), Switch/2
  Overmodulation/1 -> [Uref2], PWM Generator (3-Level)/1
  Unit Delay/1 -> [Uref1], Overmodulation/1
  "MPPT Controller using Perturbe & Observe technique "/1(D) -> Switch/1
  Switch/1 -> [Vdc_ref], VDC Regulator/2(Vdc_ref)
  Vnom_dc1/1 -> Switch/3
  Uabc_ref Generation max (m) = 1/1(Uabc_ref) -> Unit Delay/1
